simulink model "controller_abb4600"  (R2018a)
settings: Solver=FixedStepAuto  StartTime=0.0  StopTime=10.0  FixedStep=0.001  RelTol=1e-3
libraries: robotmaniplib x3
settings Model: Creator=srn  LastModifiedBy=srn
settings OptimizationCC: DefaultParameterBehavior=Inlined  EnhancedBackFolding=on  PassReuseOutputArgsAs=Individual arguments  OptimizeBlockOrder=speed  DifferentSizesBufferReuse=on  OptimizationCustomize=off
settings DebuggingCC: ParameterTunabilityLossMsg=error
settings SFSimCC: MATLABDynamicMemAlloc=off
settings RTWCC: SystemTargetFile=ert.tlc  GenCodeOnly=on  TemplateMakefile=ert_default_tmf  GenerateReport=on  IncludeHyperlinkInReport=on  LaunchReport=on  GenerateTraceInfo=on  GenerateTraceReport=on  GenerateTraceReportSl=on  GenerateTraceReportSf=on  GenerateTraceReportEml=on  GenerateCodeMetricsReport=on
settings CodeAppCC: ForceParamTrailComments=on  IgnoreCustomStorageClasses=off  OperatorAnnotations=on  SimulinkDataObjDesc=on  SFDataObjDesc=on  InsertBlockDesc=on
settings ERTTargetCC: TargetLangStandard=C99 (ISO)  GenerateSampleERTMain=on  SupportVariableSizeSignals=on  InlinedParameterPlacement=NonHierarchical  ERTCustomFileTemplate=example_file_process.tlc

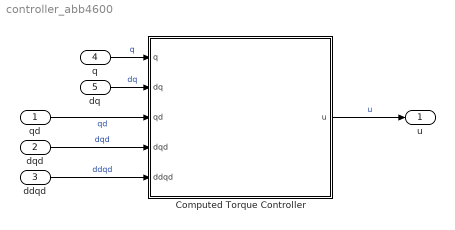
== system controller_abb4600 ==
  qd : Inport  PortDimensions=6
  dqd : Inport  Port=2  PortDimensions=6
  ddqd : Inport  Port=3  PortDimensions=6
  q : Inport  Port=4
  dq : Inport  Port=5
  Computed Torque Controller : Subsystem
  u : Outport
  wires:
  qd/1 -> Computed Torque Controller/3(qd)  "qd"
  dqd/1 -> Computed Torque Controller/4(dqd)  "dqd"
  ddqd/1 -> Computed Torque Controller/5(ddqd)  "ddqd"
  q/1 -> Computed Torque Controller/1(q)  "q"
  dq/1 -> Computed Torque Controller/2(dq)  "dq"
  Computed Torque Controller/1(u) -> u/1  "u"

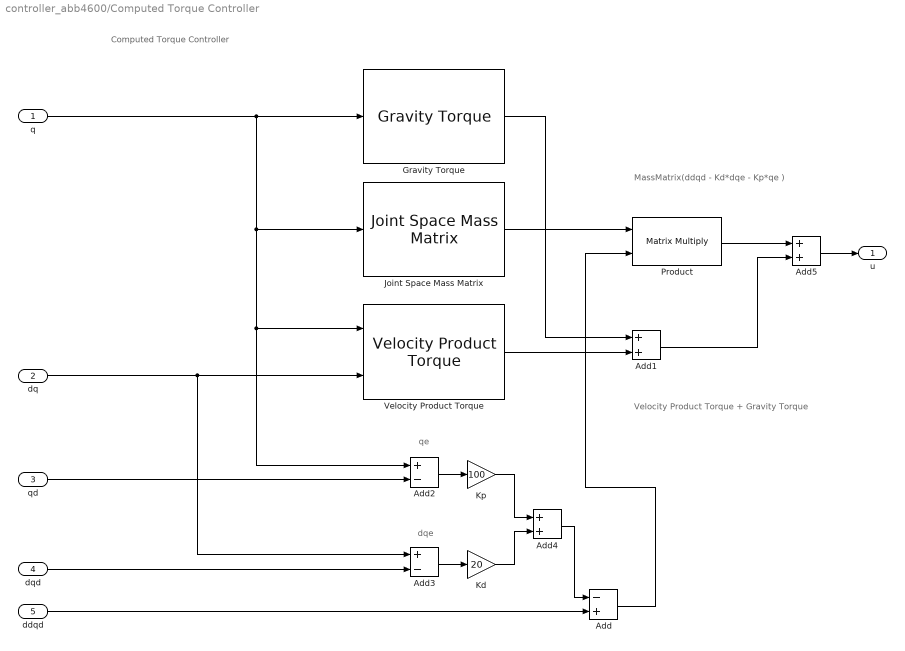
== system controller_abb4600/Computed Torque Controller ==
  note: qe
  note: dqe
  note: Velocity Product Torque + Gravity Torque
  note: MassMatrix(ddqd - Kd*dqe - Kp*qe )
  note: Computed Torque Controller
  q : Inport
  dq : Inport  Port=2
  qd : Inport  Port=3
  dqd : Inport  Port=4
  ddqd : Inport  Port=5
  Add : Sum  Inputs=-+
  Add1 : Sum
  Add2 : Sum  Inputs=+-
  Add3 : Sum  Inputs=+-
  Add4 : Sum
  Add5 : Sum
  Gravity Torque : robotmaniplib/Gravity Torque  RigidBodyTree=abb4600
      settings: SourceProductName=Robotics System Toolbox
  Joint Space Mass Matrix : robotmaniplib/Joint Space Mass Matrix  RigidBodyTree=abb4600
      settings: SourceProductName=Robotics System Toolbox
  Kd : Gain  Gain=20
  Kp : Gain  Gain=100
  Product : Product  Multiplication=Matrix(*)
  Velocity Product Torque : robotmaniplib/Velocity Product Torque  RigidBodyTree=abb4600
      settings: SourceProductName=Robotics System Toolbox
  u : Outport
  wires:
  Joint Space Mass Matrix/1 -> Product/1
  q/1 -> Gravity Torque/1, Joint Space Mass Matrix/1, Add2/1, Velocity Product Torque/1
  dq/1 -> Velocity Product Torque/2, Add3/1
  Add4/1 -> Add/1
  ddqd/1 -> Add/2
  Add/1 -> Product/2
  qd/1 -> Add2/2
  dqd/1 -> Add3/2
  Add2/1 -> Kp/1
  Add3/1 -> Kd/1
  Kp/1 -> Add4/1
  Kd/1 -> Add4/2
  Add5/1 -> u/1
  Product/1 -> Add5/1
  Add1/1 -> Add5/2
  Gravity Torque/1 -> Add1/1
  Velocity Product Torque/1 -> Add1/2
